simulink model "Transformada_inversa_Park"  (R2023b)
settings: Solver=VariableStepAuto  StartTime=0.0  StopTime=10.0  FixedStep=1e-5  RelTol=1e-3
settings Model: Creator=Julya  LastModifiedBy=Julya

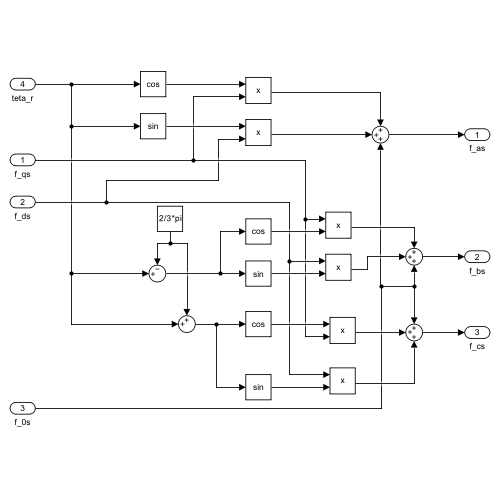
[thumbnail: Simulink's stored preview of the top-level diagram]
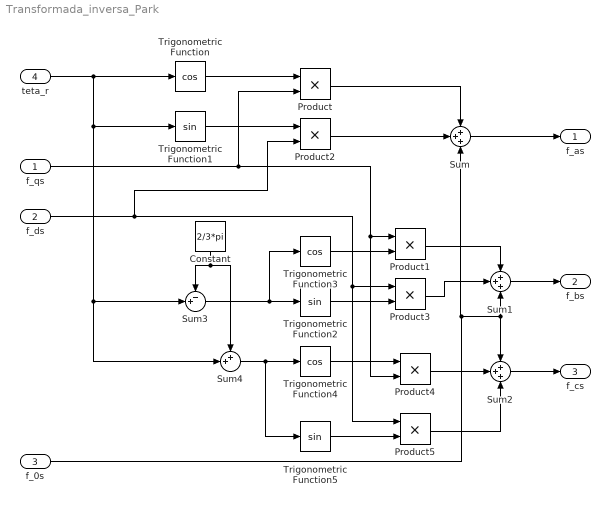
== system Transformada_inversa_Park ==
  f_qs : Inport
  f_ds : Inport  Port=2
  f_0s : Inport  Port=3
  teta_r : Inport  Port=4
  Constant : Constant  Value=2/3*pi
  Product{,1..5} (6 alike) : Product
  Sum : Sum  Inputs=+++
  Sum1 : Sum  Inputs=+++
  Sum2 : Sum  Inputs=+++
  Sum3 : Sum  Inputs=-+|
  Sum4 : Sum  Inputs=++|
  Trigonometric Function : Trigonometry  Operator=cos
  Trigonometric Function1 : Trigonometry
  Trigonometric Function2 : Trigonometry
  Trigonometric Function3 : Trigonometry  Operator=cos
  Trigonometric Function4 : Trigonometry  Operator=cos
  Trigonometric Function5 : Trigonometry
  f_as : Outport
  f_bs : Outport  Port=2
  f_cs : Outport  Port=3
  wires:
  teta_r/1 -> Sum4/2, Sum3/2, Trigonometric Function1/1, Trigonometric Function/1
  Trigonometric Function/1 -> Product/1
  f_qs/1 -> Product1/1, Product4/2, Product/2
  Trigonometric Function1/1 -> Product2/1
  f_ds/1 -> Product3/1, Product5/1, Product2/2
  Product/1 -> Sum/1
  Product2/1 -> Sum/2
  f_0s/1 -> Sum/3, Sum2/1, Sum1/3
  Sum/1 -> f_as/1
  Constant/1 -> Sum4/1, Sum3/1
  Sum3/1 -> Trigonometric Function3/1, Trigonometric Function2/1
  Sum4/1 -> Trigonometric Function5/1, Trigonometric Function4/1
  Sum1/1 -> f_bs/1
  Sum2/1 -> f_cs/1
  Trigonometric Function5/1 -> Product5/2
  Trigonometric Function3/1 -> Product1/2
  Trigonometric Function2/1 -> Product3/2
  Trigonometric Function4/1 -> Product4/1
  Product1/1 -> Sum1/1
  Product3/1 -> Sum1/2
  Product4/1 -> Sum2/2
  Product5/1 -> Sum2/3
